simulink model "Lab_Identification"  (R2021a)
settings: Solver=FixedStepAuto  StartTime=0.0  StopTime=0.1  FixedStep=1e-5  RelTol=1e-3
libraries: fl_lib x8, nesl_utility x7, ee_lib x2
settings Model: Creator=USER  LastModifiedBy=mluser

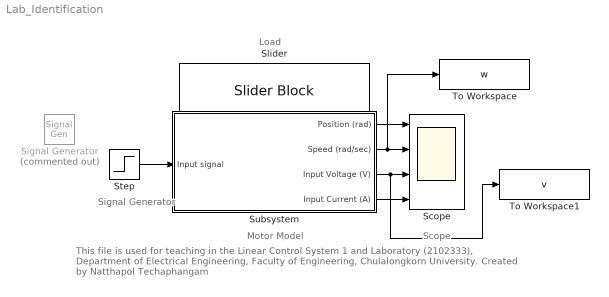
== system Lab_Identification ==
  note: This file is used for teaching in the Linear Control System 1 and Laboratory (2102333), Department of Electrical Engineering, Faculty of Engineering, Chulalongkorn University.
      |
      | Created by Natthapol Techaphangam
  note: Scope
  note: Motor Model
  note: Signal
      | Generator
  note: Load
  Scope : Scope  NumInputPorts=4
  Signal Generator : SignalGenerator  Commented=on  WaveForm=square  Amplitude=220  Frequency=100  Units=rad/sec
  Slider : SliderBlock  LabelPosition=Hide  ScaleMax=1
  Step : Step  Time=0  After=220  SampleTime=0
  Subsystem : Subsystem
  To Workspace : ToWorkspace  VariableName=w  SampleTime=-1
  To Workspace1 : ToWorkspace  VariableName=v  SampleTime=-1
  wires:
  Subsystem/4(Input Current (A)) -> Scope/4
  Subsystem/3(Input Voltage (V)) -> To Workspace1/1, Scope/3
  Subsystem/2(Speed (rad/sec)) -> To Workspace/1, Scope/2
  Subsystem/1(Position (rad)) -> Scope/1
  Step/1 -> Subsystem/1(Input signal)

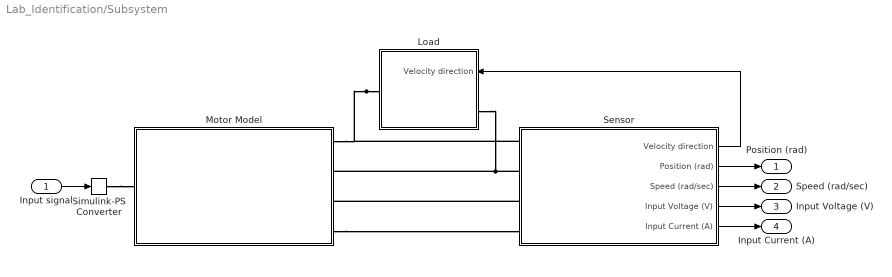
== system Lab_Identification/Subsystem ==
  Input signal : Inport
  Load : Subsystem
      settings: PortSchema="{\"entries\":[{\"content\":{\"sides\":[{\"content\":{\"connectorIds\":[\"LConn1\"]},\"type\":\"ConnectorPlacement.EquallySpacedRectSide\",\"uuid\":\"5416d762-b5b2-4cd3-a973-2cde8c761dd3\"},{\"content\":{\"connectorIds\":[\"In1\",\"RConn1\"],\"side\":\"RIGHT\"},\"type\":\"ConnectorPlacement.EquallySpacedRectSide\",\"uuid\":\"fc966553-0c06-413c-be72-9c3df9306d9c\"},{\"content\":{\"connectorIds\":[],\"side\":\"TOP\"},\"type\":\"ConnectorPlacement.EquallySpacedRectSide\",\"uuid\":\"7f121b36-502c-4a3d-8ae7-8462887c1100\"}]},\"type\":\"ConnectorPlacement.EquallySpacedConnector\",\"uuid\":\"db7ec60b-3592-4cc6-b770-272096fba341\"}],\"packageUris\":[\"http://schema.mathworks.com/mf0/Connector/R2020b\"],\"version\":\"1.0\"}"
  Motor Model : Subsystem
  Sensor : Subsystem
  Simulink-PS Converter : nesl_utility/Simulink-PS Converter  PhysicalDomain=network_engine_domain  SubClassName=ps_input  LeftPortType=input  RightPortType=output  PseudoPeriodic=off  Frequencies=[]  NoiseDistribution=none  NoiseParameters=[]  Unit=1  AffineConversion=off  FilteringAndDerivatives=provide  SimscapeFilterOrder=1  InputFilterTimeConstant=0.001  UdotUserProvided=0
      settings: SourceProductBaseCode=PW,SS
  Position (rad) : Outport
  Speed (rad/sec) : Outport  Port=2
  Input Voltage (V) : Outport  Port=3
  Input Current (A) : Outport  Port=4
  wires:
  Sensor/4(Input Voltage (V)) -> Input Voltage (V)/1
  Sensor/3(Speed (rad/sec)) -> Speed (rad/sec)/1
  Sensor/2(Position (rad)) -> Position (rad)/1
  Sensor/5(Input Current (A)) -> Input Current (A)/1
  Sensor/1(Velocity direction) -> Load/1(Velocity direction)
  Input signal/1 -> Simulink-PS Converter/1
  connections:
  Sensor/LConn2 -- Motor Model/LConn2 -- Load/RConn1
  Load/LConn1 -- Sensor/LConn1 -- Motor Model/LConn1
  Simulink-PS Converter/RConn1 -- Motor Model/RConn1
  Motor Model/LConn4 -- Sensor/LConn4
  Sensor/LConn3 -- Motor Model/LConn3

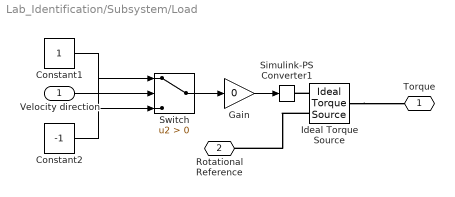
== system Lab_Identification/Subsystem/Load ==
  Velocity direction : Inport
  Constant1 : Constant
  Constant2 : Constant  Value=-1
  Gain : Gain  Gain=0
  Ideal Torque Source : fl_lib/Mechanical/Mechanical Sources/Ideal Torque Source
  Simulink-PS Converter1 : nesl_utility/Simulink-PS Converter  PhysicalDomain=network_engine_domain  SubClassName=ps_input  LeftPortType=input  RightPortType=output  PseudoPeriodic=off  Frequencies=[]  NoiseDistribution=none  NoiseParameters=[]  Unit=1  AffineConversion=off  FilteringAndDerivatives=provide  SimscapeFilterOrder=1  InputFilterTimeConstant=0.001  UdotUserProvided=0
      settings: SourceProductBaseCode=PW,SS
  Switch : Switch  Criteria=u2 > Threshold
  Torque : PMIOPort  Side=Left
  Rotational Reference : PMIOPort  Port=2  Side=Right
  wires:
  Gain/1 -> Simulink-PS Converter1/1
  Constant2/1 -> Switch/1
  Constant1/1 -> Switch/3
  Switch/1 -> Gain/1
  Velocity direction/1 -> Switch/2
  connections:
  Ideal Torque Source/RConn1 -- Simulink-PS Converter1/RConn1
  Ideal Torque Source/RConn2 -- Rotational Reference/RConn1
  Ideal Torque Source/LConn1 -- Torque/RConn1

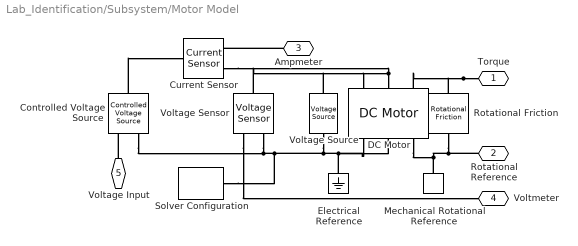
== system Lab_Identification/Subsystem/Motor Model ==
  Controlled Voltage Source : fl_lib/Electrical/Electrical Sources/Controlled Voltage Source
  Current Sensor : fl_lib/Electrical/Electrical Sensors/Current Sensor
  DC Motor : ee_lib/Electromechanical/Brushed Motors/DC Motor  field_option=ee.enum.field_option.wound  Rf=358 Ohm  Lf=2.55 H  Laf=0.15 H  If0=0 A  parameterization=ee.enum.dcparam_option.circuit_param  Ra=11.4 Ohm  La=31 mH  emf_or_torque=ee.enum.emf_or_torque.kv  Kv=0.0772 V/(rad/s)  Ki=6.876e-4 N*m/A  T_stall=0.24e-3 N*m  w_max=19100 rpm  w_rated=15000 rpm  P_rated=0.08 W  V_rated=1.5 V  J=5 g*cm^2  lam_param=ee.enum.lam_param.damping  lam=0.0035 N*m/(rad/s)  i_noload=0 A  V_i_noload=1.5 V  speed0=0 rpm  enable_fault_armature=ee.enum.faults.faultEnable.no  rev_faulted=1 / 3  G_faulted_armature=1e-5 S  fault_trigger_armature=ee.enum.faults.faultTrigger.temporal  t_fault_armature=1 s  max_permissible_current_armature=inf A  t_fail_on_current_armature=1 s  enable_fault_field=ee.enum.faults.faultEnable.no  G_faulted_field=1e-5 S  fault_trigger_field=ee.enum.faults.faultTrigger.temporal  t_fault_field=1 s  max_permissible_current_field=inf A  t_fail_on_current_field=1 s  fault_action=ee.enum.faults.faultAction.none  alpha=3.93e-3 1/K  Tmeas=25 degC  thermal_mass=100 J/K  initial_temperature=25 degC
      settings: InternalSimscapePortConfiguration="{\"Bottom\":[],\"Left\":[{\"id\":\"fp\",\"label\":\"F+\",\"type\":\"foundation.electrical.electrical\"},{\"id\":\"p\",\"label\":\"+\",\"type\":\"foundation.electrical.electrical\"},{\"id\":\"R\",\"label\":\"R\",\"type\":\"foundation.mechanical.rotational.rotational\"}],\"Right\":[{\"id\":\"fn\",\"label\":\"F-\",\"type\":\"foundation.electrical.electrical\"},{\"id\":\"n\",\"label\":\"-\",\"type\":\"foundation.electrical.electrical\"},{\"id\":\"C\",\"label\":\"C\",\"type\":\"foundation.mechanical.rotational.rotational\"}],\"Top\":[]}"
  Electrical Reference : fl_lib/Electrical/Electrical Elements/Electrical Reference
  Mechanical Rotational Reference : fl_lib/Mechanical/Rotational Elements/Mechanical Rotational Reference
  Rotational Friction : fl_lib/Mechanical/Rotational Elements/Rotational Friction  brkwy_trq=0.0005 N*m  brkwy_vel=0.0002 rad/s  Col_trq=0.0001 N*m  visc_coef=0.001 N*m/(rad/s)  w_specify=off  w_priority=None  w=0 rad/s  w_nominal_specify=off  w_nominal_unit=rad/s  w_nominal_value=1  t_specify=off  t_priority=None  t=0 N*m  t_nominal_specify=off  t_nominal_unit=N*m  t_nominal_value=1
  Solver Configuration : nesl_utility/Solver Configuration  PhysicalDomain=network_engine_domain  SubClassName=solver  LeftPortType=input  RightPortType=generic  Tones=[]  Harmonics=[]  SimulateNoise=off  Profile=off  UseLocalSampling=off  EnableSwitchedLinearOptims=on  FrequencyDomain=off  UseCCode=off  RelTol=0.001  AbsTol=1e-06  MinStep=1e-09  ToWorkspace=off  RevertToSquareIcSolve=off  NumHomotopyIterations=100  PhasorMode=off  PhasorModeNumHarmonics=1  DoDC=off  ResidualTolerance=1e-09  UseLocalSolver=off  LocalSolverChoice=NE_BACKWARD_EULER_ADVANCER  LocalSolverSampleTime=0.001  DoFixedCost=off  MaxNonlinIter=3  MaxModeIter=2  ComputeImpulses=off  ImpulseIterations=2  LinearAlgebra=auto  EquationFormulation=NE_TIME_EF  DelaysMemoryBudget=1024  AutomaticFiltering=on  FilteringTimeConstant=0.001  PartitionStorageMethod=AS_NEEDED  PartitionMemoryBudget=1024  PartitionMethod=ROBUST
      settings: SourceProductBaseCode=PW,SS
  Voltage Sensor : fl_lib/Electrical/Electrical Sensors/Voltage Sensor
  Voltage Source : ee_lib/Sources/Voltage Source  dc_voltage=200 V  ac_voltage=0 V  ac_shift=0 rad  ac_frequency=60 Hz  noise_mode=0  PSD=0 V^2/Hz  repeatability=1  auto_seed=2289918682  user_seed=0  sample_time=1e-3 s  i_specify=off  i_priority=None  i=0 A  i_nominal_specify=off  i_nominal_unit=A  i_nominal_value=1  v_specify=off  v_priority=None  v=0 V  v_nominal_specify=off  v_nominal_unit=V  v_nominal_value=1
  Torque : PMIOPort  Side=Left
  Rotational Reference : PMIOPort  Port=2  Side=Left
  Ampmeter : PMIOPort  Port=3  Side=Left
  Voltmeter : PMIOPort  Port=4  Side=Left
  Voltage Input : PMIOPort  Port=5  Side=Right
  connections:
  Rotational Friction/RConn1 -- DC Motor/RConn3 -- Mechanical Rotational Reference/LConn1 -- Rotational Reference/RConn1
  Voltage Input/RConn1 -- Controlled Voltage Source/RConn1
  DC Motor/LConn2 -- Current Sensor/RConn2 -- Voltage Sensor/LConn1
  Controlled Voltage Source/RConn2 -- Voltage Sensor/RConn2 -- Solver Configuration/RConn1 -- DC Motor/RConn2 -- DC Motor/RConn1 -- Electrical Reference/LConn1 -- Voltage Source/RConn1
  Torque/RConn1 -- Rotational Friction/LConn1 -- DC Motor/LConn3
  Controlled Voltage Source/LConn1 -- Current Sensor/LConn1
  Voltage Source/LConn1 -- DC Motor/LConn1
  Voltage Sensor/RConn1 -- Voltmeter/RConn1
  Ampmeter/RConn1 -- Current Sensor/RConn1

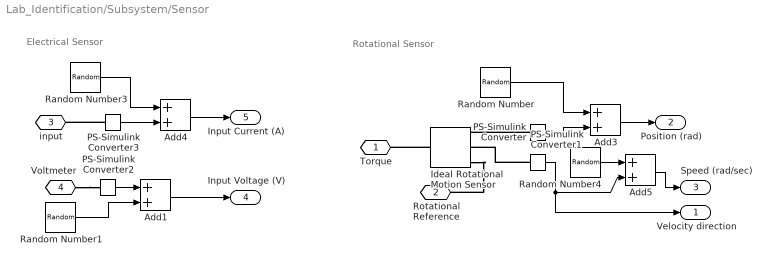
== system Lab_Identification/Subsystem/Sensor ==
  note: Rotational Sensor
  note: Electrical Sensor
  Add{1,3..5} (4 alike) : Sum
  Ideal Rotational Motion Sensor : fl_lib/Mechanical/Mechanical Sensors/Ideal Rotational Motion Sensor  wrap_angle=simscape.enum.onoff.off  offset=0 rad
  PS-Simulink Converter{,1..3} (4 alike) : nesl_utility/PS-Simulink Converter  PhysicalDomain=network_engine_domain  SubClassName=ps_output  LeftPortType=input  RightPortType=output  PseudoPeriodic=off  Frequencies=[]  Unit=inherit  AffineConversion=off
      settings: SourceProductBaseCode=PW,SS
  Random Number{,1,3..4} (4 alike) : RandomNumber  Variance=1e-3  SampleTime=1e-5
  Torque : PMIOPort  Side=Left
  Rotational Reference : PMIOPort  Port=2  Side=Left
  input : PMIOPort  Port=3  Side=Left
  Voltmeter : PMIOPort  Port=4  Side=Left
  Velocity direction : Outport
  Position (rad) : Outport  Port=2
  Speed (rad/sec) : Outport  Port=3
  Input Voltage (V) : Outport  Port=4
  Input Current (A) : Outport  Port=5
  wires:
  PS-Simulink Converter/1 -> Add3/2
  PS-Simulink Converter1/1 -> Add5/2, Velocity direction/1
  PS-Simulink Converter3/1 -> Add4/2
  Random Number3/1 -> Add4/1
  Add4/1 -> Input Current (A)/1
  Random Number/1 -> Add3/1
  Add3/1 -> Position (rad)/1
  Random Number4/1 -> Add5/1
  Add5/1 -> Speed (rad/sec)/1
  PS-Simulink Converter2/1 -> Add1/1
  Random Number1/1 -> Add1/2
  Add1/1 -> Input Voltage (V)/1
  connections:
  PS-Simulink Converter/LConn1 -- Ideal Rotational Motion Sensor/RConn3
  PS-Simulink Converter1/LConn1 -- Ideal Rotational Motion Sensor/RConn2
  Ideal Rotational Motion Sensor/LConn1 -- Torque/RConn1
  PS-Simulink Converter3/LConn1 -- input/RConn1
  Voltmeter/RConn1 -- PS-Simulink Converter2/LConn1
  Ideal Rotational Motion Sensor/RConn1 -- Rotational Reference/RConn1
